simulink model "bucket_fft"  (R2024b)
settings: Solver=FixedStepAuto  StartTime=0.0  StopTime=inf  RelTol=1e-3  EnableMultiTasking=on
model workspace (MAT data in the model file):
  fft_len = Simulink.Parameter
  fft_len.Value = 20000
  fft_len.Complexity = 'real'
  fft_len.Dimensions = [1 1]
  fft_len.DataType = 'auto'
  num_buckets = Simulink.Parameter
  num_buckets.Value = 30
  num_buckets.Complexity = 'real'
  num_buckets.Dimensions = [1 1]
  num_buckets.DataType = 'auto'
libraries: audiosources x1, dspsnks4 x1, dspxfrm3 x1, dspvision x1
settings Model: Creator=clay  LastModifiedBy=samstep
settings SolverCC: PositivePriorityOrder=on
settings OptimizationCC: DefaultParameterBehavior=Inlined  UseDivisionForNetSlopeComputation=on  GainParamInheritBuiltInType=on  UseFloatMulNetSlope=on  InlineInvariantSignals=on  EnhancedBackFolding=on  PassReuseOutputArgsAs=Individual arguments  ZeroExternalMemoryAtStartup=off  ZeroInternalMemoryAtStartup=off  EfficientFloat2IntCast=on  MaxStackSize=200000  OptimizeBlockOrder=speed  DifferentSizesBufferReuse=on  OptimizationCustomize=off  EfficientTunableParamExpr=on
settings DebuggingCC: ParameterTunabilityLossMsg=error
settings HardwareCC: ProdBitPerLong=64  ProdLargestAtomicInteger=LongLong  ProdLargestAtomicFloat=Double  ProdLongLongMode=on  ProdHWDeviceType=ARM Compatible->ARM Cortex-A (64-bit)
settings RTWCC: Description=Embedded Coder  SystemTargetFile=ert.tlc  HardwareBoard=Raspberry Pi (64bit)  TLCOptions="-aInlineSetEventsForThisBaseRateFcn=TLC_FALSE -aSuppressMultiTaskScheduler=TLC_FALSE  -aRateBasedStepFcn=0"  TemplateMakefile=ert_default_tmf  GenerateReport=on  Toolchain=GNU GCC Embedded Linux  BuildConfiguration=Faster Runs  LaunchReport=on  GPUComputeCapability=3.5
settings CodeAppCC: ForceParamTrailComments=on  IgnoreCustomStorageClasses=off  OperatorAnnotations=on  SimulinkDataObjDesc=on  SFDataObjDesc=on  InsertBlockDesc=on
settings ERTTargetCC: CodeReplacementLibrary=ARM Cortex-A CMSIS  SupportVariableSizeSignals=on  ExtModeTransport=2  ExtModeStaticAlloc=on  ExtModeMexFile=ext_xcp  ExtModeIntrfLevel=Level2 - Open

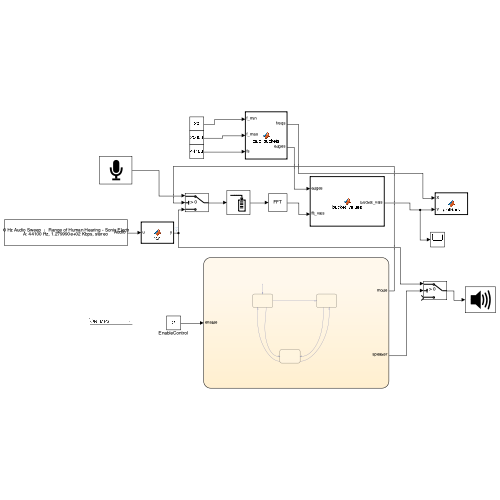
[thumbnail: Simulink's stored preview of the top-level diagram]
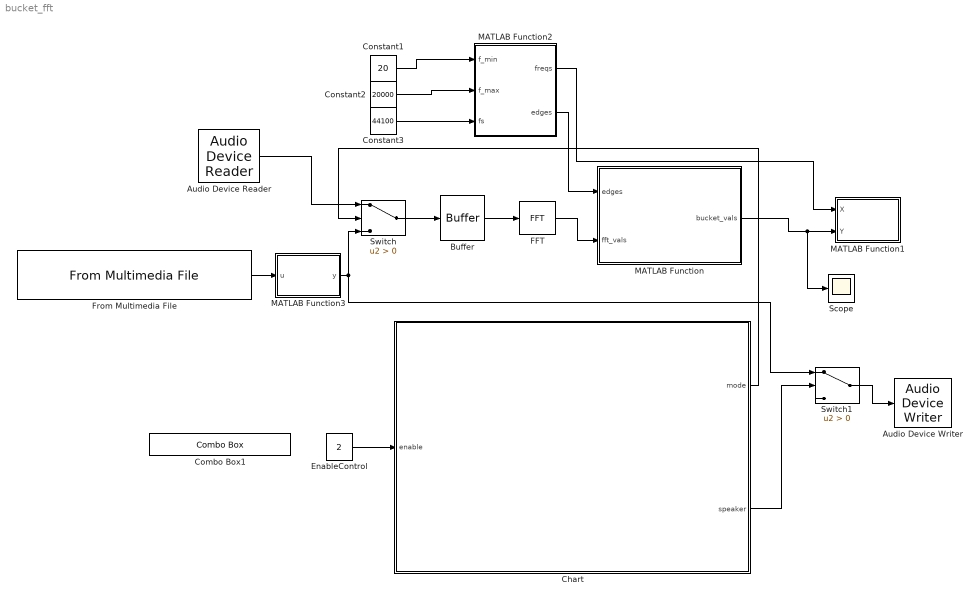
== system bucket_fft ==
  Audio Device Reader : audiosources/Audio Device Reader  Driver=CoreAudio  Device=Default  SampleRate=44100  NumChannels=1  SamplesPerFrame=1024  BitDepth=16-bit integer  NumBuffers=10  DefaultInputChannelMapping=on  InputChannelMapping=1:2  OutputNumOverrunSamples=off  OutputDataType=double  DriverIdx=5  DeviceWarnFlag=''
  Audio Device Writer : dspsnks4/Audio Device Writer  Driver=CoreAudio  Device=MacBook Pro Speakers  InheritSampleRate=on  SampleRate=44100  BitDepth=16-bit integer  BufferSize=4096  NumBuffers=10  DefaultOutputChannelMapping=on  OutputChannelMapping=1:2  OutputNumUnderrunSamples=off  DriverIdx=5  DeviceWarnFlag=''
  Buffer : Buffer  N=fft_len  V=200  OutputFrames=off
  Chart : Stateflow chart  TreatAsAtomicUnit=on
  Combo Box1 : ComboBox  LabelPosition=Hide  SelectedLabel=ON: MP3
      settings: Values={{'OFF', 'ON: Microphone', 'ON: MP3'}, [0 1 2]}
  Constant1 : Constant  Value=20
  Constant2 : Constant  Value=20000
  Constant3 : Constant  Value=44100
  EnableControl : Constant  Value=2
  FFT : dspxfrm3/FFT  FFTImplementation=Auto  CompMethod=Table lookup  TableOpt=NEW  TableOptActive=Speed  BitRevOrder=off  Normalize=off  InheritFFTLength=on  FFTLength=64  WrapInput=on  roundingMode=Floor  overflowMode=off  firstCoeffDataTypeStr=Inherit: Same word length as input  firstCoeffLastDataTypeStr=Inherit: Same word length as input  outputMin=[]  outputMax=[]
  From Multimedia File : dspvision/From Multimedia File  inputFilename=/Users/samstep/Documents/MATLAB/503/Final Project/20 - 20,000 Hz Audio Sweep ｜ Range of Human Hearing - Sonic Electronix.mp3  readRange=[1 Inf]  loop=on  numPlays=inf  outputStreams=Audio only  videoDataType=single  audioDataType=double  inheritSampleTime=on  userDefinedSampleTime=1/30  noAudioOutput=off  isIntensityVideo=off  fourcc=RGB  colorVideoFormat=Separate color signals  outputEOF=off  dataOrg=Column-major  audioFrameSize=1024  computeAudioFrameSize=off  outSamplingMode=Sample based
      settings: LibrarySourceBlock=audiosources/From Multimedia File
  MATLAB Function : MATLAB Function  TreatAsAtomicUnit=on
  MATLAB Function1 : MATLAB Function  TreatAsAtomicUnit=on
  MATLAB Function2 : MATLAB Function  TreatAsAtomicUnit=on
  MATLAB Function3 : MATLAB Function  TreatAsAtomicUnit=on
  Scope : Scope
  Switch : Switch  Criteria=u2 > Threshold  SaturateOnIntegerOverflow=off  InputSameDT=off
  Switch1 : Switch  Criteria=u2 > Threshold  SaturateOnIntegerOverflow=off  InputSameDT=off
  wires:
  Audio Device Reader/1 -> Switch/1
  Switch/1 -> Buffer/1
  Buffer/1 -> FFT/1
  FFT/1 -> MATLAB Function/2(fft_vals)
  MATLAB Function/1(bucket_vals) -> Scope/1, MATLAB Function1/2(Y)
  MATLAB Function2/2(edges) -> MATLAB Function/1(edges)
  MATLAB Function2/1(freqs) -> MATLAB Function1/1(X)
  Constant3/1 -> MATLAB Function2/3(fs)
  Constant2/1 -> MATLAB Function2/2(f_max)
  Constant1/1 -> MATLAB Function2/1(f_min)
  MATLAB Function3/1(y) -> Switch/3, Switch1/1
  EnableControl/1 -> Chart/1(enable)
  From Multimedia File/1 -> MATLAB Function3/1(u)
  Switch1/1 -> Audio Device Writer/1
  Chart/2(speaker) -> Switch1/2
  Chart/1(mode) -> Switch/2

== matlab function bucket_fft/MATLAB Function1 ==
  data: X input; Y input
function plotBars(X,Y)

coder.extrinsic('stem')
stem(X,Y)
set(gca,'xscal','log')
axis([20, 20000, 0, 300])

end

== matlab function bucket_fft/MATLAB Function ==
  data: edges input; fft_vals input; bucket_vals output
function bucket_vals  = bucket_values(edges, fft_vals)

bucket_vals = zeros(1, length(edges)-1);

for i = 1:length(edges)-1
    range = abs(fft_vals(edges(i):edges(i+1)-1));
    bucket_vals(i) = max(range);
end

% fs = 44100;
% fft_len = 1024;
% freq_edges = (edges - 1) * fs / fft_len;
% freqs = (freq_edges(1:end-1) + freq_edges(2:end)) / 2;

end

== matlab function bucket_fft/MATLAB Function2 ==
  data: freqs output; f_min input; f_max input; fs input; edges output; fft_len parameter; num_buckets parameter
function [freqs, edges] = calc_buckets(f_min, f_max, fs, fft_len, num_buckets)

% coder.const(fft_len)
% coder.const(num_buckets)

edge_min = ceil(f_min * fft_len / fs)
edge_max = floor(f_max * fft_len / fs)

edges = ceil(logspace(log10(edge_min), log10(edge_max), num_buckets + 1))
freq_edges = (edges - 1) * fs / fft_len;
freqs = (freq_edges(1:end-1) + freq_edges(2:end)) / 2;

end

== stateflow chart bucket_fft/Chart ==
  state IDLE
  state micMode
  state mp3Mode
  (default) -> IDLE : {enable==0,speaker=0,mode=0}
  IDLE -> micMode [order 1] : [enable==1]{mode=1,speaker=0}
  mp3Mode -> IDLE [order 1] : [enable==0]{speaker=0, mode=0}
  IDLE -> mp3Mode [order 2] : [enable==2]{mode=0,speaker=1}
  micMode -> mp3Mode : [enable==2]{mode=0,speaker=1}
  mp3Mode -> micMode [order 2] : [enable==1]{mode=1,speaker=0}
  data: mode output double; enable input; speaker output double

== matlab function bucket_fft/MATLAB Function3 ==
  data: u input; y output
function y = fcn(u)

y = u(:,1);
